simulink model "SG__MDL"  (R2022b)
settings: Solver=FixedStepAuto  StartTime=0.0  StopTime=Inf  FixedStep=ts  RelTol=1e-3  EnableMultiTasking=on
settings Model: SimulationMode=external  ExplicitPartitioning=on  DataflowThreadingImplementation=OpenMP  Creator=padlewsk  LastModifiedBy=padlewsk
settings SolverCC: ConcurrentTasks=on  AlgebraicLoopSolver=TrustRegion  PositivePriorityOrder=on  AutoInsertRateTranBlk=on
settings DataIOCC: SaveFormat=StructureWithTime
settings OptimizationCC: GainParamInheritBuiltInType=on  UseFloatMulNetSlope=on  RollThreshold=9  EfficientFloat2IntCast=on  SimCompilerOptimization=on
settings DebuggingCC: TasksWithSamePriorityMsg=none  UnconnectedInputMsg=warning  UnconnectedOutputMsg=warning  UnconnectedLineMsg=warning
settings HardwareCC: ProdBitPerLong=64  ProdLongLongMode=on  ProdHWDeviceType=Intel->x86-64 (Linux 64)
settings ModelReferenceCC: EnableRefExpFcnMdlSchedulingChecks=on
settings RTWCC: Description=Simulink Real-Time  SystemTargetFile=slrealtime.tlc  TemplateMakefile=slrealtime_default_tmf  Toolchain=Simulink Real-Time Toolchain  BuildConfiguration=Faster Runs  CodeExecutionProfiling=on  CodeProfilingInstrumentation=coarse  TargetLang=C++

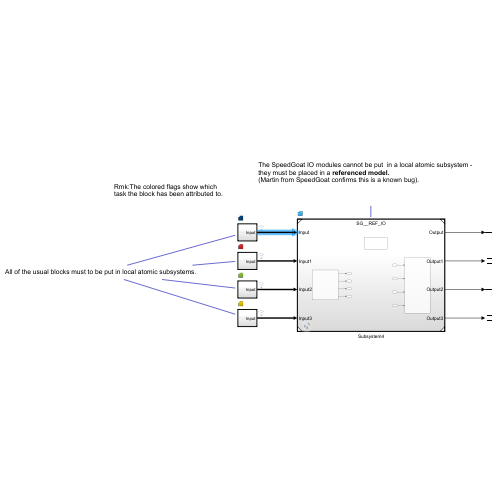
[thumbnail: Simulink's stored preview of the top-level diagram]
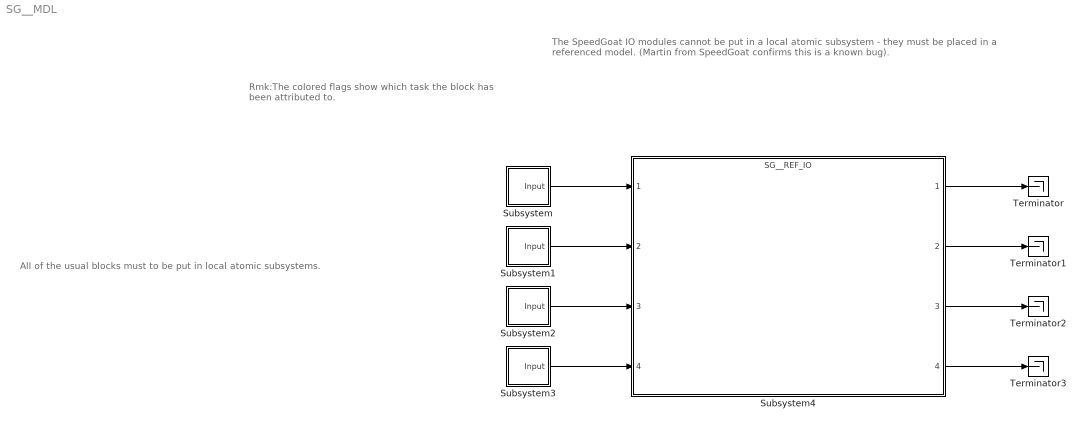
== system SG__MDL ==
  note: Rmk:The colored flags show which task the block has been attributed to.
  note: The SpeedGoat IO modules cannot be put in a local atomic subsystem - they must be placed in a referenced model.
      | (Martin from SpeedGoat confirms this is a known bug).
  note: All of the usual blocks must to be put in local atomic subsystems.
  Subsystem : Subsystem  TreatAsAtomicUnit=on
  Subsystem1 : Subsystem  TreatAsAtomicUnit=on
  Subsystem2 : Subsystem  TreatAsAtomicUnit=on
  Subsystem3 : Subsystem  TreatAsAtomicUnit=on
  Subsystem4 : ModelReference  ModelNameDialog=SG__REF_IO.slx  SimulationMode=Normal  ModelReferenceVersion=5.5
  Terminator{,1..3} (4 alike) : Terminator
  wires:
  Subsystem/1(Input) -> Subsystem4/1
  Subsystem4/1 -> Terminator/1
  Subsystem4/2 -> Terminator1/1
  Subsystem4/3 -> Terminator2/1
  Subsystem4/4 -> Terminator3/1
  Subsystem1/1(Input) -> Subsystem4/2
  Subsystem2/1(Input) -> Subsystem4/3
  Subsystem3/1(Input) -> Subsystem4/4

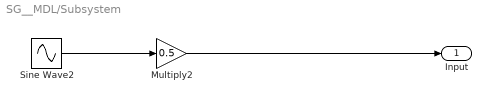
== system SG__MDL/Subsystem ==
  Multiply2 : Gain  Gain=0.5
  Sine Wave2 : Sin  Frequency=2*pi*10
  Input : Outport
  wires:
  Sine Wave2/1 -> Multiply2/1
  Multiply2/1 -> Input/1

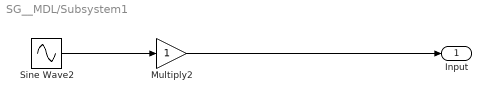
== system SG__MDL/Subsystem1 ==
  Multiply2 : Gain
  Sine Wave2 : Sin  Frequency=2*pi*10
  Input : Outport
  wires:
  Sine Wave2/1 -> Multiply2/1
  Multiply2/1 -> Input/1

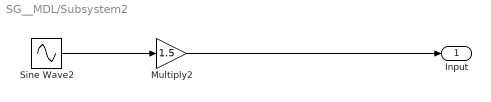
== system SG__MDL/Subsystem2 ==
  Multiply2 : Gain  Gain=1.5
  Sine Wave2 : Sin  Frequency=2*pi*10
  Input : Outport
  wires:
  Sine Wave2/1 -> Multiply2/1
  Multiply2/1 -> Input/1

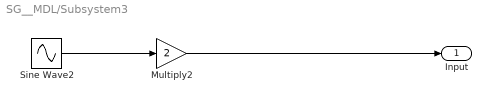
== system SG__MDL/Subsystem3 ==
  Multiply2 : Gain  Gain=2
  Sine Wave2 : Sin  Frequency=2*pi*10
  Input : Outport
  wires:
  Sine Wave2/1 -> Multiply2/1
  Multiply2/1 -> Input/1
